simulink model "simfile_assignment_02"  (R2024a)
settings: Solver=VariableStepAuto  StartTime=0.0  StopTime=10.0  RelTol=1e-3
values from neighbouring files (symbols this model uses):
  A = input("enter the value for A: \n")    [mscript_assignment_02.m]
  F = input("enter the value of F: \n")    [mscript_assignment_02.m]
  Ti = input("enter the value for Ti: \n")    [mscript_assignment_02.m]
settings Model: Creator=admin  LastModifiedBy=admin

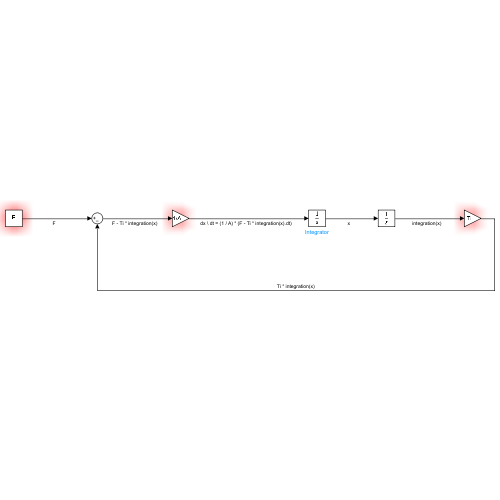
[thumbnail: Simulink's stored preview of the top-level diagram]
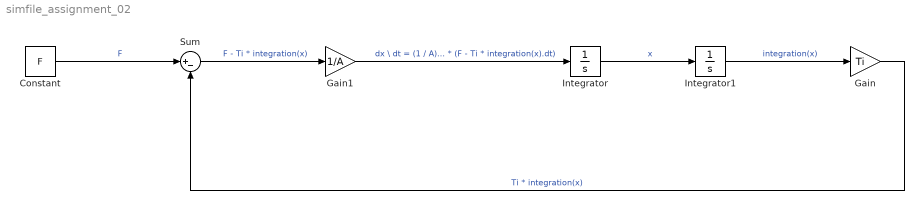
== system simfile_assignment_02 ==
  Constant : Constant  Value=F
  Gain : Gain  Gain=Ti
  Gain1 : Gain  Gain=1/A
  Integrator : Integrator
  Integrator1 : Integrator
  Sum : Sum  Inputs=|+-
  wires:
  Integrator/1 -> Integrator1/1  "x"
  Sum/1 -> Gain1/1  "F - Ti * integration(x)"
  Integrator1/1 -> Gain/1  "integration(x)"
  Gain/1 -> Sum/2  "Ti * integration(x)"
  Constant/1 -> Sum/1  "F"
  Gain1/1 -> Integrator/1  "dx \\ dt = (1 / A) * (F - Ti * integration(x).dt)"
